simulink model "untitled2"  (R2023a)
settings: Solver=VariableStepAuto  StartTime=0.0  StopTime=10.0  RelTol=1e-3
undefined symbols (not defined in the file): g, k, l
libraries: matrix_library x1
settings Model: Creator=abi7287  LastModifiedBy=abi7287

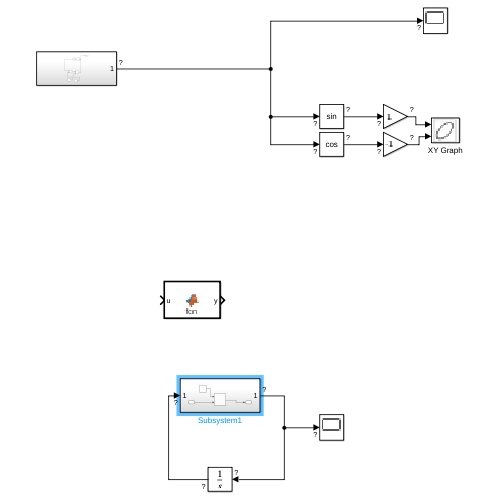
[thumbnail: Simulink's stored preview of the top-level diagram]
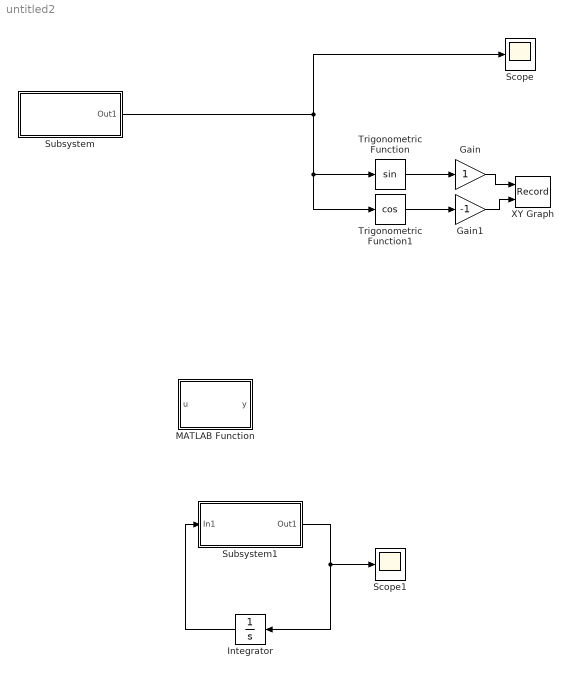
== system untitled2 ==
  Gain : Gain
  Gain1 : Gain  Gain=-1
  Integrator : Integrator
  MATLAB Function : MATLAB Function  TreatAsAtomicUnit=on
  Scope : Scope
  Scope1 : Scope
  Subsystem : Subsystem
  Subsystem1 : Subsystem
  Trigonometric Function : Trigonometry
  Trigonometric Function1 : Trigonometry  Operator=cos
  XY Graph : Record  FileSettingsInternal="{\"entries\":[{\"content\":{\"excelSettings\":{\"content\":{},\"type\":\"Streamout.ExcelSettings\"}},\"type\":\"Streamout.FileSettingStorage\",\"uuid\":\"229df6fc-c6f0-45a3-b438-1a3f9e4f6bfe\"}],\"packageUris\":[\"http://schema.mathworks.com/mf0/streamout_blocks/R2020a\"],\"version\":\"1.0\"}"  Layout=[1 1]  SignalsInternal="{\"entries\":[{\"content\":{\"signals\":[{\"content\":{\"blockPath\":[\"untitled2/XY Graph\"],\"dimensions\":[1],\"domain\":\"untitled2/XY Graph\",\"lineColor\":\"#a2142f\",\"plots\":[1],\"port\":1,\"signalID\":75,\"signalName\":\"XY Graph:1\"},\"type\":\"RecordBlkView.Signal\",\"uuid\":\"f74d12c6-3b75-4576-901e-74475d7cef89\"},{\"content\":{\"blockPath\":[\"untitled2/XY Graph\"],\"dimensions\":[1],\"domain\":\"untitled2/XY Graph\",\"lineColor\":\"#139fff\",\"plots\":[1],\"port\":2,\"signalID\":78,\"signalName\":\"XY Graph:2\"},\"type\":\"RecordBlkView.Signal\",\"uuid\":\"26390821-0b74-4bb2-8100-2862ec3848cd\"}]},\"type\":\"RecordBlkView.InputSignals\",\"uuid\":\"aea6ec99-2f8a-41c4-836d-9d0115e5b773\"}],\"packageUris\":[\"http://schema.mathworks.com/mf0/streamout_blocks/R2020a\"],\"version\":\"1.0\"}"  VisualizationBindings="{\"xyplotplugin\":{\"info\":[{\"series\":[{\"bindingParametersList\":[{\"parameter\":\"X-Axis\",\"signalID\":75,\"signalName\":\"XY Graph:1\"},{\"parameter\":\"Y-Axis\",\"signalID\":78,\"signalName\":\"XY Graph:2\"}],\"seriesID\":60439}],\"subplotID\":1}]}}"  CompatibilityTag=XY
  wires:
  Subsystem/1(Out1) -> Scope/1, Trigonometric Function1/1, Trigonometric Function/1
  Gain/1 -> XY Graph/1
  Gain1/1 -> XY Graph/2
  Trigonometric Function/1 -> Gain/1
  Trigonometric Function1/1 -> Gain1/1
  Integrator/1 -> Subsystem1/1(In1)
  Subsystem1/1(Out1) -> Scope1/1, Integrator/1

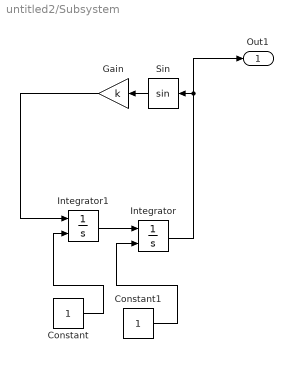
== system untitled2/Subsystem ==
  Constant : Constant
  Constant1 : Constant
  Gain : Gain  Gain=k
  Integrator : Integrator  InitialConditionSource=external  InitialCondition=1
  Integrator1 : Integrator  InitialConditionSource=external  InitialCondition=1
  Sin : Trigonometry
  Out1 : Outport
  wires:
  Sin/1 -> Gain/1
  Constant/1 -> Integrator1/2
  Constant1/1 -> Integrator/2
  Integrator/1 -> Out1/1, Sin/1
  Integrator1/1 -> Integrator/1
  Gain/1 -> Integrator1/1

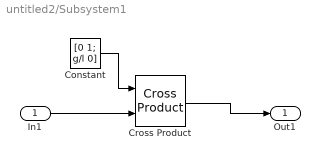
== system untitled2/Subsystem1 ==
  In1 : Inport
  Constant : Constant  Value=[0 1; g/l 0]
  Cross Product : matrix_library/Cross Product
  Out1 : Outport
  wires:
  Constant/1 -> Cross Product/1
  Cross Product/1 -> Out1/1
  In1/1 -> Cross Product/2

== matlab function untitled2/MATLAB Function ==
  data: u input; y output
function y = fcn(u)

y = u;
